simulink model "NandiniG_23EEM1S02_bldc_foc"  (R2024b)
settings: Solver=VariableStepAuto  StartTime=0.0  StopTime=1  FixedStep=0.000001  MaxStep=1e-4  RelTol=1e-3
model workspace (MAT data in the model file):
  fs = 4000
undefined symbols (not defined in the file): Ts
libraries: simulink x13, spsIGBTDiodeLib x6, slpidlib x3, spsPermanentMagnetSynchronousMachineLib x1, spsDCVoltageSourceLib x1, spsSawtoothGeneratorLib x1, simulink_extras x1, spsThreePhaseVIMeasurementLib x1, spspowerguiLib x1
settings Model: Creator=Admin  LastModifiedBy=INNAGOL2
settings SolverCC: ZeroCrossAlgorithm=Adaptive
settings DebuggingCC: MaskedZcDiagnostic=none  IgnoredZcDiagnostic=none
settings RTWCC: GPUComputeCapability=3.5

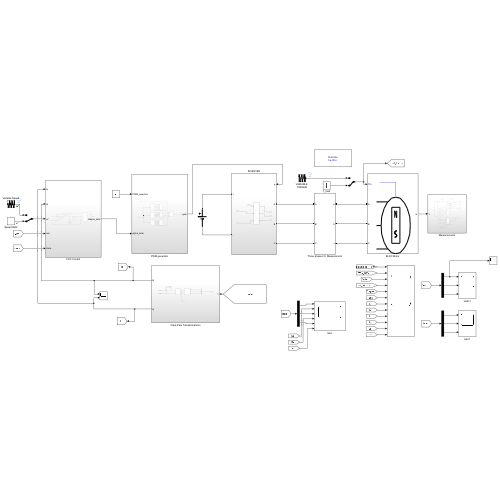
[thumbnail: Simulink's stored preview of the top-level diagram]
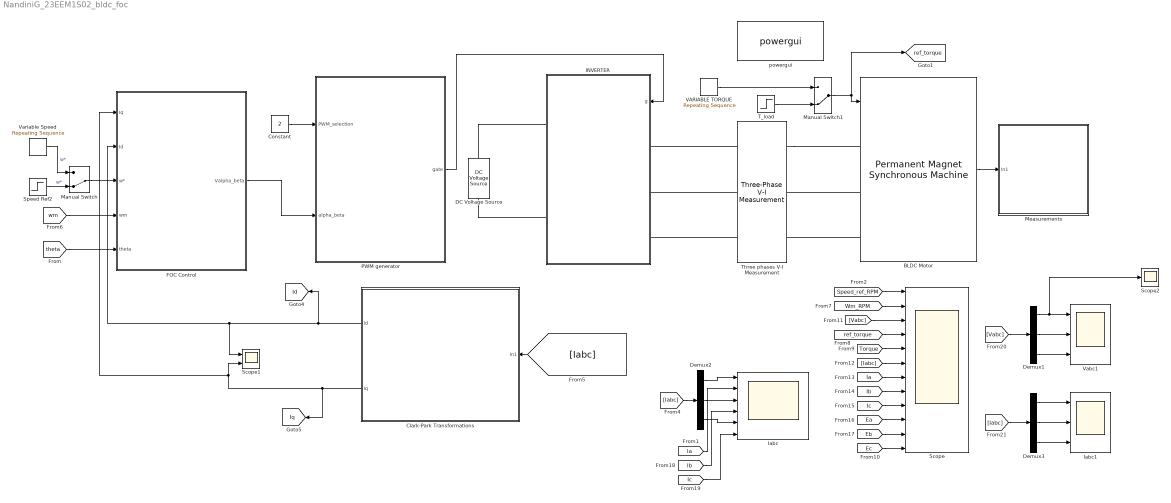
== system NandiniG_23EEM1S02_bldc_foc ==
  BLDC Motor : spsPermanentMagnetSynchronousMachineLib/Permanent Magnet Synchronous Machine  NbPhases=3  FluxDistribution=Trapezoidal  RotorType=Round  MechanicalLoad=Torque Tm  PresetModel=No  ShowDetailedParameters=on  MeasurementBus=off  Resistance=0.7  Inductance=2.7e-3  dqInductances=[8.5e-3,8.5e-3]  La=0.000835  MachineConstant=Flux linkage established by magnets (V.s)  Flux=0.1194  VoltageCst=100.0283  TorqueCst=0.9552  Flat=120  Mechanical=[0.0027 0.0004924 4]  PolePairs=4  InitialConditions=[0,0, 0,0]  InitialConditions5ph=[0 0 0 0 0 0]  RefAngle=Aligned with phase A axis (original Park)  IterativeDiscreteModel=Trapezoidal non iterative  TsBlock=-1  TsPowergui=0
  Clark-Park Transformations : Subsystem
      settings: PortSchema="{\"entries\":[{\"content\":{\"sides\":[{\"content\":{\"connectorIds\":[\"Out1\",\"Out2\"]},\"type\":\"ConnectorPlacement.EquallySpacedRectSide\",\"uuid\":\"c290a13d-b4ce-440f-9d53-4b9274feb83f\"},{\"content\":{\"connectorIds\":[\"In1\"],\"side\":\"RIGHT\"},\"type\":\"ConnectorPlacement.EquallySpacedRectSide\",\"uuid\":\"3b8acf4d-0134-48df-ade6-fa9dd8548719\"},{\"content\":{\"side\":\"TOP\"},\"type\":\"ConnectorPlacement.EquallySpacedRectSide\",\"uuid\":\"08682ee2-bcb7-4f48-a64a-1997ed6d0a04\"}]},\"type\":\"ConnectorPlacement.EquallySpacedConnector\",\"uuid\":\"e640fd84-78ba-4bab-8695-1c4b1b64123a\"}],\"packageUris\":[\"http://schema.mathworks.com/mf0/Connector/R2020b\"],\"version\":\"1.0\"}"
  Constant : Constant  Value=2
  DC Voltage Source : spsDCVoltageSourceLib/DC Voltage Source  Amplitude=160  Measurements=None
  Demux1 : Demux  Outputs=3
  Demux2 : Demux  Outputs=3
  Demux3 : Demux  Outputs=3
  FOC Control : Subsystem
  INVERTER : Subsystem
  Iabc : Scope  NumInputPorts=6
  Iabc1 : Scope  NumInputPorts=3
  Manual Switch : ManualSwitch  CurrentSetting=0
  Manual Switch1 : ManualSwitch  CurrentSetting=0
  Measurements : Subsystem
  PWM generator : Subsystem
  Scope : Scope  NumInputPorts=12
  Scope1 : Scope  NumInputPorts=2
  Scope2 : Scope
  Speed Ref2 : Step  Time=0.1  After=150  SampleTime=0
  "T_load " : Step  Time=0.1  After=5  SampleTime=0
  Three phases V-I Measurement : spsThreePhaseVIMeasurementLib/Three-Phase V-I Measurement  VoltageMeasurement=phase-to-phase  SetLabelV=on  LabelV=Vabc  Vpu=off  VpuLL=off  CurrentMeasurement=yes  SetLabelI=on  LabelI=Iabc  Ipu=off  Pbase=100e6  Vbase=500e3  OutputType=Complex  PhasorSimulation=off  PSBequivalent=0
  VARIABLE TORQUE : simulink/Sources/Repeating Sequence  rep_seq_t=[0 1 2 3 4 5 6 7 8 9 10 11 12 13]  rep_seq_y=[3 3 3 3 5 5 5 -2 -2 -2 1 1 1 1 ]
  Vabc1 : Scope  NumInputPorts=3
  Variable Speed : simulink/Sources/Repeating Sequence  rep_seq_t=[0 1 2 3 4 5 6 7 8 9 10 11 11.0001 12 13]  rep_seq_y=[0 20 20 0 0 0 -30 -30 0 0 50 50 40 40 0]
  powergui : spspowerguiLib/powergui  Priority=1  SimulationMode=Discrete  SampleTime=5e-05  frequency=60  Iterations=50  frequencyindice=0  Pbase=100e6  ErrMax=1e-4  UnitsV=kV  UnitsW=MW  buscounter=0  FunctionMessages=off  echomessages=off  EnableUseOfTLC=off  CurrentSourceSwitches=off  DisableSnubberDevices=off  DisableRonSwitches=off  DisableVfSwitches=off  DisplayEquations=off  AutomaticDiscreteSolvers=off  SolverType=Tustin/Backward Euler (TBE)  Interpol=off  ExternalGateDelay=off  methode=off  Ts=100  x0status=blocks  SPID=on  SwTol=0  HookPort=off  NonlinearTolerance=1e-4  nMaxIteration=100  ContinueOnMaxIteration=off  RestoreLinks=warning  ResistiveCurrentMeasurement=off  Frange=[0:2:500]  Ylog=off  Xlog=on  ShowGrid=off  save=off  variable=ZData  structure=0  ZoomFFT=off  StartTime=0.0  cycles=1  DisplayStyle=1  fundamental=60  FreqAxis=off  MaxFrequency=1000  frequencyindicesteady=1  RmsSteady=1  display=off
  tag scope: Id=global, Iq=global, ref_torque=global
  wires:
  Demux2/1 -> Iabc/1
  Demux2/2 -> Iabc/3
  Demux2/3 -> Iabc/5
  [Iabc] -> Demux2/1
  PWM generator/1(gate) -> INVERTER/1(g)
  [Iabc] -> Clark-Park Transformations/1(In1)
  Clark-Park Transformations/1(Id) -> Scope1/1, FOC Control/2(Id), [Id]
  Clark-Park Transformations/2(Iq) -> Scope1/2, FOC Control/1(Iq), [Iq]
  [wm] -> FOC Control/4(wm)
  [theta] -> FOC Control/5(theta)
  Constant/1 -> PWM generator/1(PWM_selection)
  FOC Control/1(Valpha_beta) -> PWM generator/2(alpha_beta)
  Speed Ref2/1 -> Manual Switch/2  "w*"
  Manual Switch/1 -> FOC Control/3(w*)
  VARIABLE TORQUE/1 -> Manual Switch1/1
  "T_load "/1 -> Manual Switch1/2
  Manual Switch1/1 -> BLDC Motor/1, [ref_torque]
  Variable Speed/1 -> Manual Switch/1  "w*"
  BLDC Motor/1 -> Measurements/1(In1)
  [Vabc] -> Scope/3
  [Ib] -> Scope/8
  [Ia] -> Scope/7
  [Ea] -> Scope/10
  [ref_torque] -> Scope/4
  [Ic] -> Scope/9
  [Ec] -> Scope/12
  [Eb] -> Scope/11
  [Torque] -> Scope/5
  [Wm_RPM] -> Scope/2
  [Iabc] -> Scope/6
  [Speed_ref_RPM] -> Scope/1
  [Ia] -> Iabc/2
  [Ib] -> Iabc/4
  [Ic] -> Iabc/6
  Demux1/2 -> Vabc1/2
  Demux3/2 -> Iabc1/2
  [Vabc] -> Demux1/1
  Demux3/3 -> Iabc1/3
  Demux1/1 -> Scope2/1, Vabc1/1
  Demux1/3 -> Vabc1/3
  Demux3/1 -> Iabc1/1
  [Iabc] -> Demux3/1
  connections:
  BLDC Motor/LConn2 -- Three phases V-I Measurement/RConn2
  BLDC Motor/LConn3 -- Three phases V-I Measurement/RConn3
  Three phases V-I Measurement/LConn1 -- INVERTER/LConn1
  DC Voltage Source/RConn1 -- INVERTER/RConn1
  Three phases V-I Measurement/LConn2 -- INVERTER/LConn2
  DC Voltage Source/LConn1 -- INVERTER/RConn2
  Three phases V-I Measurement/LConn3 -- INVERTER/LConn3
  Three phases V-I Measurement/RConn1 -- BLDC Motor/LConn1

== system NandiniG_23EEM1S02_bldc_foc/Clark-Park Transformations ==
  In1 : Inport
  Clark Transformation : Subsystem
  Demux1 : Demux  Outputs=3
  Park Transformation : Subsystem
  Scope3 : Scope  NumInputPorts=2
  Id : Outport
  Iq : Outport  Port=2
  wires:
  Park Transformation/2(Iq) -> Iq/1, Scope3/2  "Iq"
  Demux1/1 -> Clark Transformation/1(Ia)
  Park Transformation/1(Id) -> Id/1, Scope3/1  "Id"
  [theta] -> Park Transformation/3(theta)
  Demux1/2 -> Clark Transformation/2(Ib)
  Clark Transformation/2(I_beta) -> Park Transformation/2(I_beta)
  Demux1/3 -> Clark Transformation/3(Ic)
  Clark Transformation/1(I_alpha) -> Park Transformation/1(I_alpha)
  In1/1 -> Demux1/1

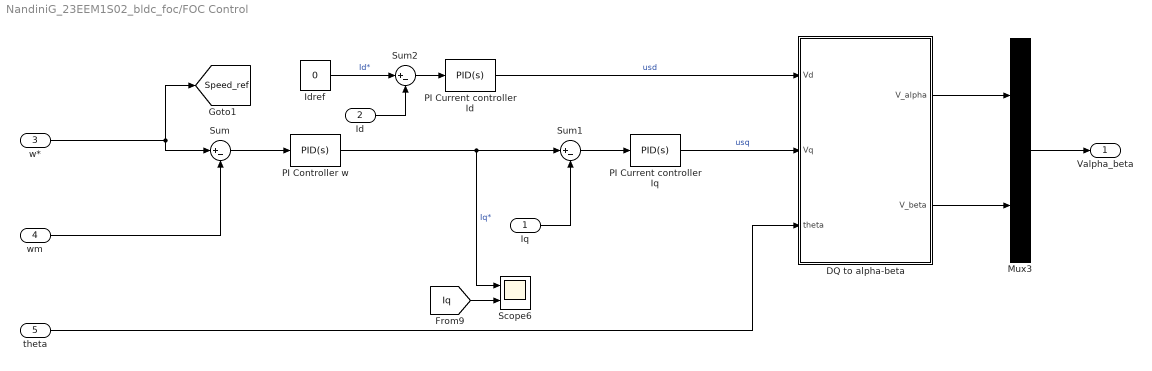
== system NandiniG_23EEM1S02_bldc_foc/FOC Control ==
  Iq : Inport
  Id : Inport  Port=2
  w* : Inport  Port=3
  wm : Inport  Port=4
  theta : Inport  Port=5
  DQ to alpha-beta : Subsystem
  Idref : Constant  Value=0
  Mux3 : Mux  Inputs=2
  PI Controller w : slpidlib/PID Controller  Controller=PID  Form=Parallel  TimeDomain=Continuous-time  UseExternalTs=off  SampleTime=-1  IntegratorMethod=Forward Euler  FilterMethod=Forward Euler  ControllerParametersSource=internal  P=18  I=35  UseKiTs=off  D=0  UseExternalDerivativeSource=off  N=100  UseFilter=on  TunerSelectOption=Frequency Response Based  InitialConditionSource=internal  InitialConditionForIntegrator=0  InitialConditionForFilter=0  DifferentiatorICPrevScaledInput=0  ExternalReset=none  TrackingMode=off  Kt=1  LimitOutput=on  SatLimitsSource=internal  UpperSaturationLimit=60  LowerSaturationLimit=-60  LinearizeAsGain=on  AntiWindupMode=none  Kb=1  LimitIntegrator=on  UpperIntegratorSaturationLimit=60  LowerIntegratorSaturationLimit=-60  POutMin=[]  POutMax=[]  IOutMin=[]  IOutMax=[]  DOutMin=[]  DOutMax=[]  NOutMin=[]  NOutMax=[]  SumOutMin=[]  SumOutMax=[]  SaturationOutMin=[]  SaturationOutMax=[]  PParamMin=[]  PParamMax=[]  IParamMin=[]  IParamMax=[]  DParamMin=[]  DParamMax=[]  NParamMin=[]  NParamMax=[]  KbParamMin=[]  KbParamMax=[]  KtParamMin=[]  KtParamMax=[]  KbOutMin=[]  KbOutMax=[]  KtOutMin=[]  KtOutMax=[]  IntegratorOutMin=[]  IntegratorOutMax=[]  FilterOutMin=[]  FilterOutMax=[]  SumI1OutMin=[]  SumI1OutMax=[]  SumI2OutMin=[]  SumI2OutMax=[]  SumI3OutMin=[]  SumI3OutMax=[]  SumI4OutMin=[]  SumI4OutMax=[]  SumDOutMin=[]  SumDOutMax=[]  DifferentiatorOutMin=[]  DifferentiatorOutMax=[]  FilterDiffOutCoefMin=[]  FilterDiffOutCoefMax=[]  ReciprocalOutMin=[]  ReciprocalOutMax=[]  SumDenOutMin=[]  SumDenOutMax=[]  SumNumOutMin=[]  SumNumOutMax=[]  DivideOutMin=[]  DivideOutMax=[]  UdiffTsProdOutMin=[]  UdiffTsProdOutMax=[]  NTsProdOutMin=[]  NTsProdOutMax=[]  UintegralTsProdOutMin=[]  UintegralTsProdOutMax=[]  UngainTsProdOutMin=[]  UngainTsProdOutMax=[]  ClampingZeroOutDataTypeStr=Inherit: Inherit via back propagation  ClampingZeroOutMin=[]  ClampingZeroOutMax=[]  FilterDenConstantOutDataTypeStr=Inherit: Inherit via back propagation  FilterDenConstantOutMin=[]  FilterDenConstantOutMax=[]  PCopyOutDataTypeStr=Inherit: Inherit via back propagation  PCopyOutMin=[]  PCopyOutMax=[]  NCopyOutDataTypeStr=Inherit: Inherit via back propagation  NCopyOutMin=[]  NCopyOutMax=[]  IntegratorContinuousStateAttributes=''  IntegratorStateMustResolveToSignalObject=off  IntegratorRTWStateStorageClass=Auto  FilterContinuousStateAttributes=''  FilterStateMustResolveToSignalObject=off  FilterRTWStateStorageClass=Auto  ParallelPVariant=InternalParameters  IdealPVariant=Disabled  IVariant=InternalParameters  DVariant=InternalParameters  IntegratorVariant=Continuous  SatVariant=Enabled  AWVariant=Passthrough  PCopyVariant=Disabled  TRVariant=Disabled  FdbkBlocksVariant=Forward  IdealPFdbkVariant=Disabled  SatFdbkVariant=Disabled  DerivativeFilterVariant=ContFilter  NVariant=InternalParameters  NCopyVariant=Disabled  FilterICVariant=InternalICsFilter  IntegratorICVariant=InternalICs  ExternalResetVariant=Disabled  TRSumVariant=Passthrough  SumFdbkVariant=Disabled  SumVariant=Sum_PID  TsampFilterVariant=InternalTs  TsampNgainVariant=Passthrough  TsampIntegralVariant=Disabled_SignalSpec  ExternalSaturationOutDataTypeStr=Inherit: Same as second input  DerivativeSourceVariant=ErrorSignal  PreIntVariant=InternalPreInt
  PI Current controller Id : slpidlib/PID Controller  Controller=PID  Form=Parallel  TimeDomain=Continuous-time  UseExternalTs=off  SampleTime=-1  IntegratorMethod=Forward Euler  FilterMethod=Forward Euler  ControllerParametersSource=internal  P=100  I=1000  UseKiTs=off  D=0  UseExternalDerivativeSource=off  N=100  UseFilter=on  TunerSelectOption=Transfer Function Based (PID Tuner App)  InitialConditionSource=internal  InitialConditionForIntegrator=0  InitialConditionForFilter=0  DifferentiatorICPrevScaledInput=0  ExternalReset=none  TrackingMode=off  Kt=1  LimitOutput=on  SatLimitsSource=internal  UpperSaturationLimit=600  LowerSaturationLimit=-600  LinearizeAsGain=on  AntiWindupMode=clamping  Kb=1  LimitIntegrator=off  UpperIntegratorSaturationLimit=inf  LowerIntegratorSaturationLimit=-inf  POutMin=[]  POutMax=[]  IOutMin=[]  IOutMax=[]  DOutMin=[]  DOutMax=[]  NOutMin=[]  NOutMax=[]  SumOutMin=[]  SumOutMax=[]  SaturationOutMin=[]  SaturationOutMax=[]  PParamMin=[]  PParamMax=[]  IParamMin=[]  IParamMax=[]  DParamMin=[]  DParamMax=[]  NParamMin=[]  NParamMax=[]  KbParamMin=[]  KbParamMax=[]  KtParamMin=[]  KtParamMax=[]  KbOutMin=[]  KbOutMax=[]  KtOutMin=[]  KtOutMax=[]  IntegratorOutMin=[]  IntegratorOutMax=[]  FilterOutMin=[]  FilterOutMax=[]  SumI1OutMin=[]  SumI1OutMax=[]  SumI2OutMin=[]  SumI2OutMax=[]  SumI3OutMin=[]  SumI3OutMax=[]  SumI4OutMin=[]  SumI4OutMax=[]  SumDOutMin=[]  SumDOutMax=[]  DifferentiatorOutMin=[]  DifferentiatorOutMax=[]  FilterDiffOutCoefMin=[]  FilterDiffOutCoefMax=[]  ReciprocalOutMin=[]  ReciprocalOutMax=[]  SumDenOutMin=[]  SumDenOutMax=[]  SumNumOutMin=[]  SumNumOutMax=[]  DivideOutMin=[]  DivideOutMax=[]  UdiffTsProdOutMin=[]  UdiffTsProdOutMax=[]  NTsProdOutMin=[]  NTsProdOutMax=[]  UintegralTsProdOutMin=[]  UintegralTsProdOutMax=[]  UngainTsProdOutMin=[]  UngainTsProdOutMax=[]  ClampingZeroOutDataTypeStr=Inherit: Inherit via back propagation  ClampingZeroOutMin=[]  ClampingZeroOutMax=[]  FilterDenConstantOutDataTypeStr=Inherit: Inherit via back propagation  FilterDenConstantOutMin=[]  FilterDenConstantOutMax=[]  PCopyOutDataTypeStr=Inherit: Inherit via back propagation  PCopyOutMin=[]  PCopyOutMax=[]  NCopyOutDataTypeStr=Inherit: Inherit via back propagation  NCopyOutMin=[]  NCopyOutMax=[]  IntegratorContinuousStateAttributes=''  IntegratorStateMustResolveToSignalObject=off  IntegratorRTWStateStorageClass=Auto  FilterContinuousStateAttributes=''  FilterStateMustResolveToSignalObject=off  FilterRTWStateStorageClass=Auto  ParallelPVariant=InternalParameters  IdealPVariant=Disabled  IVariant=InternalParameters  DVariant=InternalParameters  IntegratorVariant=Continuous  SatVariant=Enabled  AWVariant=ContClampingParallel  PCopyVariant=Disabled  TRVariant=Disabled  FdbkBlocksVariant=Forward  IdealPFdbkVariant=Disabled  SatFdbkVariant=Disabled  DerivativeFilterVariant=ContFilter  NVariant=InternalParameters  NCopyVariant=Disabled  FilterICVariant=InternalICsFilter  IntegratorICVariant=InternalICs  ExternalResetVariant=Disabled  TRSumVariant=Passthrough  SumFdbkVariant=Disabled  SumVariant=Sum_PID  TsampFilterVariant=InternalTs  TsampNgainVariant=Passthrough  TsampIntegralVariant=Disabled_SignalSpec  ExternalSaturationOutDataTypeStr=Inherit: Same as second input  DerivativeSourceVariant=ErrorSignal  PreIntVariant=InternalPreInt
  PI Current controller Iq : slpidlib/PID Controller  Controller=PID  Form=Parallel  TimeDomain=Continuous-time  UseExternalTs=off  SampleTime=-1  IntegratorMethod=Forward Euler  FilterMethod=Forward Euler  ControllerParametersSource=internal  P=100  I=1000  UseKiTs=off  D=0  UseExternalDerivativeSource=off  N=100  UseFilter=on  TunerSelectOption=Transfer Function Based (PID Tuner App)  InitialConditionSource=internal  InitialConditionForIntegrator=0  InitialConditionForFilter=0  DifferentiatorICPrevScaledInput=0  ExternalReset=none  TrackingMode=off  Kt=1  LimitOutput=on  SatLimitsSource=internal  UpperSaturationLimit=600  LowerSaturationLimit=-600  LinearizeAsGain=on  AntiWindupMode=clamping  Kb=1  LimitIntegrator=off  UpperIntegratorSaturationLimit=inf  LowerIntegratorSaturationLimit=-inf  POutMin=[]  POutMax=[]  IOutMin=[]  IOutMax=[]  DOutMin=[]  DOutMax=[]  NOutMin=[]  NOutMax=[]  SumOutMin=[]  SumOutMax=[]  SaturationOutMin=[]  SaturationOutMax=[]  PParamMin=[]  PParamMax=[]  IParamMin=[]  IParamMax=[]  DParamMin=[]  DParamMax=[]  NParamMin=[]  NParamMax=[]  KbParamMin=[]  KbParamMax=[]  KtParamMin=[]  KtParamMax=[]  KbOutMin=[]  KbOutMax=[]  KtOutMin=[]  KtOutMax=[]  IntegratorOutMin=[]  IntegratorOutMax=[]  FilterOutMin=[]  FilterOutMax=[]  SumI1OutMin=[]  SumI1OutMax=[]  SumI2OutMin=[]  SumI2OutMax=[]  SumI3OutMin=[]  SumI3OutMax=[]  SumI4OutMin=[]  SumI4OutMax=[]  SumDOutMin=[]  SumDOutMax=[]  DifferentiatorOutMin=[]  DifferentiatorOutMax=[]  FilterDiffOutCoefMin=[]  FilterDiffOutCoefMax=[]  ReciprocalOutMin=[]  ReciprocalOutMax=[]  SumDenOutMin=[]  SumDenOutMax=[]  SumNumOutMin=[]  SumNumOutMax=[]  DivideOutMin=[]  DivideOutMax=[]  UdiffTsProdOutMin=[]  UdiffTsProdOutMax=[]  NTsProdOutMin=[]  NTsProdOutMax=[]  UintegralTsProdOutMin=[]  UintegralTsProdOutMax=[]  UngainTsProdOutMin=[]  UngainTsProdOutMax=[]  ClampingZeroOutDataTypeStr=Inherit: Inherit via back propagation  ClampingZeroOutMin=[]  ClampingZeroOutMax=[]  FilterDenConstantOutDataTypeStr=Inherit: Inherit via back propagation  FilterDenConstantOutMin=[]  FilterDenConstantOutMax=[]  PCopyOutDataTypeStr=Inherit: Inherit via back propagation  PCopyOutMin=[]  PCopyOutMax=[]  NCopyOutDataTypeStr=Inherit: Inherit via back propagation  NCopyOutMin=[]  NCopyOutMax=[]  IntegratorContinuousStateAttributes=''  IntegratorStateMustResolveToSignalObject=off  IntegratorRTWStateStorageClass=Auto  FilterContinuousStateAttributes=''  FilterStateMustResolveToSignalObject=off  FilterRTWStateStorageClass=Auto  ParallelPVariant=InternalParameters  IdealPVariant=Disabled  IVariant=InternalParameters  DVariant=InternalParameters  IntegratorVariant=Continuous  SatVariant=Enabled  AWVariant=ContClampingParallel  PCopyVariant=Disabled  TRVariant=Disabled  FdbkBlocksVariant=Forward  IdealPFdbkVariant=Disabled  SatFdbkVariant=Disabled  DerivativeFilterVariant=ContFilter  NVariant=InternalParameters  NCopyVariant=Disabled  FilterICVariant=InternalICsFilter  IntegratorICVariant=InternalICs  ExternalResetVariant=Disabled  TRSumVariant=Passthrough  SumFdbkVariant=Disabled  SumVariant=Sum_PID  TsampFilterVariant=InternalTs  TsampNgainVariant=Passthrough  TsampIntegralVariant=Disabled_SignalSpec  ExternalSaturationOutDataTypeStr=Inherit: Same as second input  DerivativeSourceVariant=ErrorSignal  PreIntVariant=InternalPreInt
  Scope6 : Scope  NumInputPorts=2
  Sum : Sum  Inputs=|+-
  Sum1 : Sum  Inputs=|+-
  Sum2 : Sum  Inputs=|+-
  Valpha_beta : Outport
  tag scope: Speed_ref=global
  wires:
  PI Current controller Iq/1 -> DQ to alpha-beta/2(Vq)  "usq"
  PI Controller w/1 -> Scope6/1, Sum1/1  "Iq*"
  theta/1 -> DQ to alpha-beta/3(theta)
  Idref/1 -> Sum2/1  "Id*"
  Sum1/1 -> PI Current controller Iq/1
  Sum2/1 -> PI Current controller Id/1
  Sum/1 -> PI Controller w/1
  w*/1 -> [Speed_ref], Sum/1
  [Iq] -> Scope6/2
  PI Current controller Id/1 -> DQ to alpha-beta/1(Vd)  "usd"
  DQ to alpha-beta/1(V_alpha) -> Mux3/1
  DQ to alpha-beta/2(V_beta) -> Mux3/2
  Mux3/1 -> Valpha_beta/1
  Iq/1 -> Sum1/2
  wm/1 -> Sum/2
  Id/1 -> Sum2/2

== system NandiniG_23EEM1S02_bldc_foc/INVERTER ==
  g : Inport
  Subsystem1 : Subsystem
  A : PMIOPort  Side=Left
  B : PMIOPort  Port=2  Side=Left
  C : PMIOPort  Port=3  Side=Left
  + : PMIOPort  Port=4  Side=Right
  - : PMIOPort  Port=5  Side=Right
  wires:
  g/1 -> Subsystem1/1(Gate)
  connections:
  C/RConn1 -- Subsystem1/RConn3
  B/RConn1 -- Subsystem1/RConn2
  A/RConn1 -- Subsystem1/RConn1
  +/RConn1 -- Subsystem1/LConn1
  -/RConn1 -- Subsystem1/LConn2

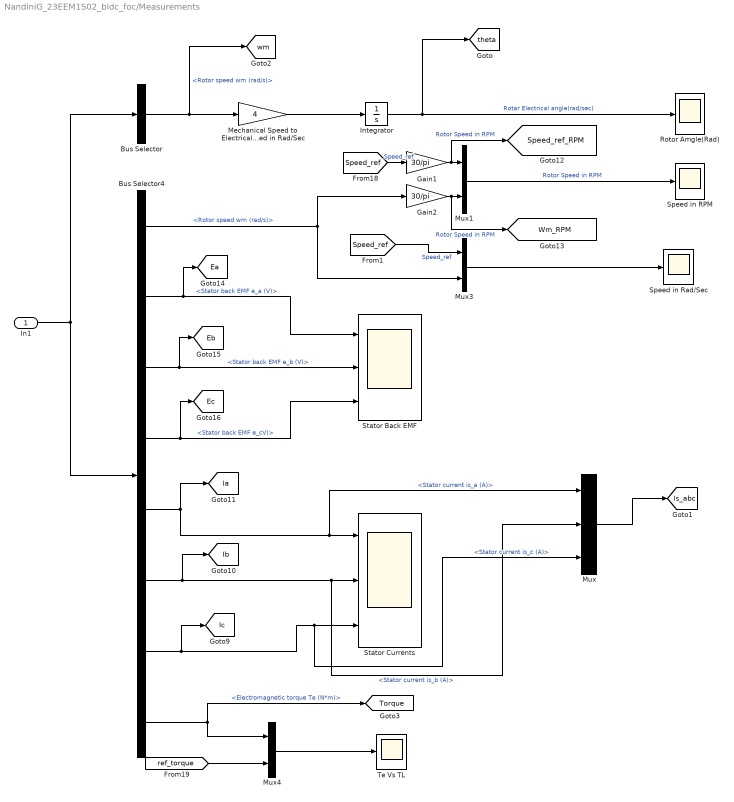
== system NandiniG_23EEM1S02_bldc_foc/Measurements ==
  In1 : Inport
  Bus Selector : BusSelector  OutputSignals=Rotor speed wm (rad/s)
  Bus Selector4 : BusSelector  OutputSignals=Rotor speed wm (rad/s),Stator back EMF e_a (V),Stator back EMF e_b (V),Stator back EMF e_cV),Stator current is_a (A),Stator current is_b (A),Stator current is_c (A),Electromagnetic torque Te (N*m)
  Gain1 : Gain  Gain=30/pi
  Gain2 : Gain  Gain=30/pi
  Integrator : Integrator  WrapState=on
  Mechanical Speed to Electrical speed in Rad/Sec : Gain  Gain=4
  Mux : Mux  Inputs=3
  Mux1 : Mux  Inputs=2
  Mux3 : Mux  Inputs=2
  Mux4 : Mux  Inputs=2
  Rotor Amgle(Rad) : Scope
  Speed in RPM : Scope
  Speed in Rad/Sec : Scope
  Stator Back EMF : Scope  NumInputPorts=3
  Stator Currents : Scope  NumInputPorts=3
  Te Vs TL : Scope
  tag scope: Ea=global, Eb=global, Ec=global, Ia=global, Ib=global, Ic=global, Is_abc=global, Speed_ref_RPM=global, Torque=global, Wm_RPM=global, theta=global, wm=global
  wires:
  [ref_torque] -> Mux4/2
  Mechanical Speed to Electrical speed in Rad/Sec/1 -> Integrator/1
  Mux4/1 -> Te Vs TL/1
  Bus Selector/1 -> [wm], Mechanical Speed to Electrical speed in Rad/Sec/1  "<Rotor speed wm (rad/s)>"
  Bus Selector4/3 -> [Eb], Stator Back EMF/2  "<Stator back EMF e_b (V)>"
  Bus Selector4/8 -> [Torque], Mux4/1  "<Electromagnetic torque Te (N*m)>"
  Bus Selector4/5 -> [Ia], Mux/1, Stator Currents/1  "<Stator current is_a (A)>"
  In1/1 -> Bus Selector4/1, Bus Selector/1
  Bus Selector4/4 -> [Ec], Stator Back EMF/3  "<Stator back EMF e_cV)>"
  Gain2/1 -> [Wm_RPM], Mux1/2  "Rotor Speed in RPM"
  Bus Selector4/7 -> [Ic], Mux/3, Stator Currents/3  "<Stator current is_c (A)>"
  Integrator/1 -> [theta], Rotor Amgle(Rad)/1  "Rotar Electrical angle(rad/sec)"
  Bus Selector4/2 -> [Ea], Stator Back EMF/1  "<Stator back EMF e_a (V)>"
  Bus Selector4/1 -> Mux3/2, Gain2/1  "<Rotor speed wm (rad/s)>"
  Gain1/1 -> [Speed_ref_RPM], Mux1/1  "Rotor Speed in RPM"
  Mux3/1 -> Speed in Rad/Sec/1
  Mux1/1 -> Speed in RPM/1  "Rotor Speed in RPM"
  [Speed_ref] -> Gain1/1  "Speed_ref"
  Bus Selector4/6 -> [Ib], Mux/2, Stator Currents/2  "<Stator current is_b (A)>"
  [Speed_ref] -> Mux3/1  "Speed_ref"
  Mux/1 -> [Is_abc]

== system NandiniG_23EEM1S02_bldc_foc/PWM generator ==
  PWM_selection : Inport
  alpha_beta : Inport  Port=2
  Gate : Scope  NumInputPorts=6
  Multiport Switch : MultiPortSwitch  SaturateOnIntegerOverflow=off  InputSameDT=off
  PWM : Subsystem
  SPWM : Subsystem
  SVPWM : Subsystem
  Scope4 : Scope  NumInputPorts=6
  Scope9 : Scope  NumInputPorts=6
  gate : Outport
  wires:
  SVPWM/2(g4) -> Scope9/2
  PWM/2(g4) -> Scope4/2
  PWM/3(g3) -> Scope4/3
  PWM/1(g1) -> Scope4/1
  SPWM/3(g3) -> Gate/3
  SVPWM/1(g1) -> Scope9/1
  alpha_beta/1 -> SPWM/1(alpha_beta), SVPWM/1(alpha beta), PWM/1(alpha_beta)
  SVPWM/3(g3) -> Scope9/3
  PWM/5(g5) -> Scope4/5
  PWM/7(Gate) -> Multiport Switch/4
  PWM/6(g2) -> Scope4/6
  SPWM/5(g5) -> Gate/5
  SPWM/4(g6) -> Gate/4
  SPWM/1(g1) -> Gate/1
  SPWM/2(g4) -> Gate/2
  SPWM/6(g2) -> Gate/6
  SPWM/7(gate) -> Multiport Switch/2
  PWM/4(g6) -> Scope4/4
  PWM_selection/1 -> Multiport Switch/1
  Multiport Switch/1 -> gate/1
  SVPWM/4(g6) -> Scope9/4
  SVPWM/5(g5) -> Scope9/5
  SVPWM/6(g2) -> Scope9/6
  SVPWM/7(Gate1) -> Multiport Switch/3

== system NandiniG_23EEM1S02_bldc_foc/Clark-Park Transformations/Clark Transformation ==
  Ia : Inport
  Ib : Inport  Port=2
  Ic : Inport  Port=3
  Gain : Gain
  Gain1 : Gain  Gain=-1/2
  Gain2 : Gain  Gain=-1/2
  Gain3 : Gain  Gain=(sqrt(3))/2
  Gain4 : Gain  Gain=(-sqrt(3))/2
  Sum3 : Sum  Inputs=|+++
  Sum4 : Sum  Inputs=|++
  I_alpha : Outport
  I_beta : Outport  Port=2
  wires:
  Gain2/1 -> Sum3/3
  Ib/1 -> Gain3/1, Gain1/1
  Sum3/1 -> I_alpha/1
  Gain3/1 -> Sum4/1
  Gain/1 -> Sum3/1
  Ic/1 -> Gain4/1, Gain2/1
  Gain1/1 -> Sum3/2
  Gain4/1 -> Sum4/2
  Ia/1 -> Gain/1
  Sum4/1 -> I_beta/1

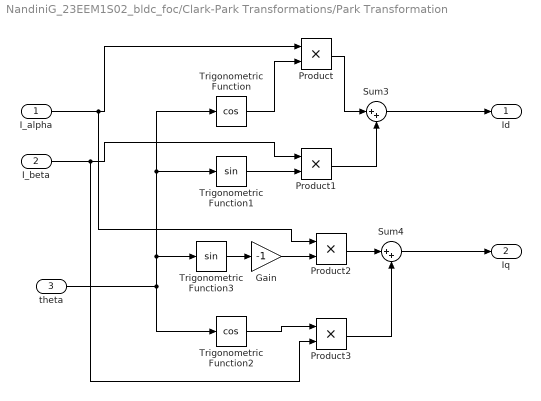
== system NandiniG_23EEM1S02_bldc_foc/Clark-Park Transformations/Park Transformation ==
  I_alpha : Inport
  I_beta : Inport  Port=2
  theta : Inport  Port=3
  Gain : Gain  Gain=-1
  Product{,1..3} (4 alike) : Product
  Sum3 : Sum  Inputs=|++
  Sum4 : Sum  Inputs=|++
  Trigonometric Function : Trigonometry  Operator=cos
  Trigonometric Function1 : Trigonometry
  Trigonometric Function2 : Trigonometry  Operator=cos
  Trigonometric Function3 : Trigonometry
  Id : Outport
  Iq : Outport  Port=2
  wires:
  Sum3/1 -> Id/1
  Sum4/1 -> Iq/1
  Trigonometric Function3/1 -> Gain/1
  theta/1 -> Trigonometric Function2/1, Trigonometric Function3/1, Trigonometric Function1/1, Trigonometric Function/1
  Trigonometric Function/1 -> Product/2
  I_alpha/1 -> Product2/1, Product/1
  Trigonometric Function1/1 -> Product1/2
  I_beta/1 -> Product3/2, Product1/1
  Product/1 -> Sum3/1
  Product1/1 -> Sum3/2
  Gain/1 -> Product2/2
  Trigonometric Function2/1 -> Product3/1
  Product2/1 -> Sum4/1
  Product3/1 -> Sum4/2

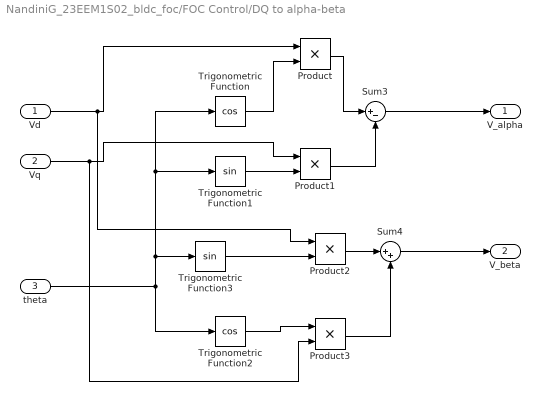
== system NandiniG_23EEM1S02_bldc_foc/FOC Control/DQ to alpha-beta ==
  Vd : Inport
  Vq : Inport  Port=2
  theta : Inport  Port=3
  Product{,1..3} (4 alike) : Product
  Sum3 : Sum  Inputs=|+-
  Sum4 : Sum  Inputs=|++
  Trigonometric Function : Trigonometry  Operator=cos
  Trigonometric Function1 : Trigonometry
  Trigonometric Function2 : Trigonometry  Operator=cos
  Trigonometric Function3 : Trigonometry
  V_alpha : Outport
  V_beta : Outport  Port=2
  wires:
  Product3/1 -> Sum4/2
  Product2/1 -> Sum4/1
  Trigonometric Function2/1 -> Product3/1
  Trigonometric Function3/1 -> Product2/2
  Product1/1 -> Sum3/2
  Product/1 -> Sum3/1
  Vq/1 -> Product1/1, Product3/2
  Trigonometric Function1/1 -> Product1/2
  Vd/1 -> Product/1, Product2/1
  Trigonometric Function/1 -> Product/2
  theta/1 -> Trigonometric Function/1, Trigonometric Function1/1, Trigonometric Function3/1, Trigonometric Function2/1
  Sum4/1 -> V_beta/1
  Sum3/1 -> V_alpha/1

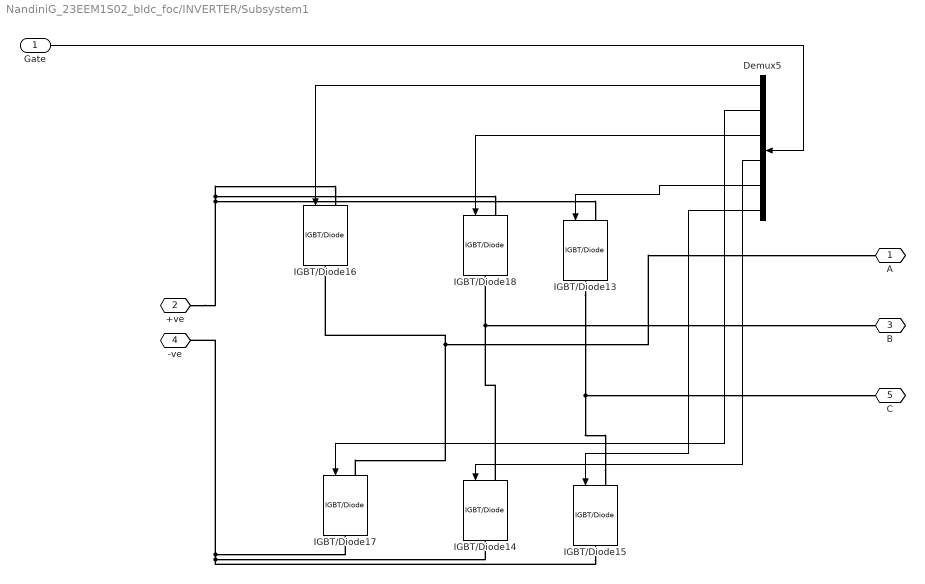
== system NandiniG_23EEM1S02_bldc_foc/INVERTER/Subsystem1 ==
  Gate : Inport
  Demux5 : Demux  Outputs=6
  IGBT/Diode{13..18} (6 alike) : spsIGBTDiodeLib/IGBT//Diode  Ron=1e-3  Rs=1e5  Cs=inf  Measurements=off
  A : PMIOPort  Side=Right
  +ve : PMIOPort  Port=2  Side=Left
  B : PMIOPort  Port=3  Side=Right
  -ve : PMIOPort  Port=4  Side=Left
  C : PMIOPort  Port=5  Side=Right
  wires:
  Demux5/3 -> IGBT/Diode18/1
  Demux5/2 -> IGBT/Diode17/1
  Demux5/6 -> IGBT/Diode15/1
  Demux5/1 -> IGBT/Diode16/1
  Gate/1 -> Demux5/1
  Demux5/4 -> IGBT/Diode14/1
  Demux5/5 -> IGBT/Diode13/1
  connections:
  IGBT/Diode15/LConn1 -- C/RConn1 -- IGBT/Diode13/RConn1
  IGBT/Diode18/RConn1 -- B/RConn1 -- IGBT/Diode14/LConn1
  IGBT/Diode14/RConn1 -- IGBT/Diode17/RConn1 -- -ve/RConn1 -- IGBT/Diode15/RConn1
  IGBT/Diode16/RConn1 -- A/RConn1 -- IGBT/Diode17/LConn1
  IGBT/Diode16/LConn1 -- IGBT/Diode18/LConn1 -- +ve/RConn1 -- IGBT/Diode13/LConn1

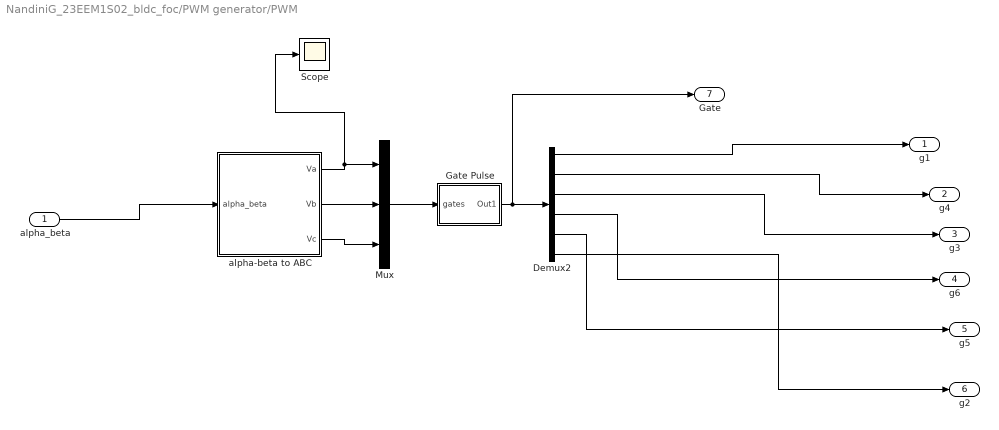
== system NandiniG_23EEM1S02_bldc_foc/PWM generator/PWM ==
  alpha_beta : Inport
  Demux2 : Demux  Outputs=6
  Gate Pulse : Subsystem
  Mux : Mux  Inputs=3
  Scope : Scope
  alpha-beta to ABC : Subsystem
  g1 : Outport
  g4 : Outport  Port=2
  g3 : Outport  Port=3
  g6 : Outport  Port=4
  g5 : Outport  Port=5
  g2 : Outport  Port=6
  Gate : Outport  Port=7
  wires:
  Gate Pulse/1(Out1) -> Gate/1, Demux2/1
  alpha-beta to ABC/3(Vc) -> Mux/3
  Demux2/3 -> g3/1
  alpha-beta to ABC/1(Va) -> Scope/1, Mux/1
  Mux/1 -> Gate Pulse/1(gates)
  Demux2/5 -> g5/1
  Demux2/2 -> g4/1
  alpha-beta to ABC/2(Vb) -> Mux/2
  alpha_beta/1 -> alpha-beta to ABC/1(alpha_beta)
  Demux2/6 -> g2/1
  Demux2/4 -> g6/1
  Demux2/1 -> g1/1

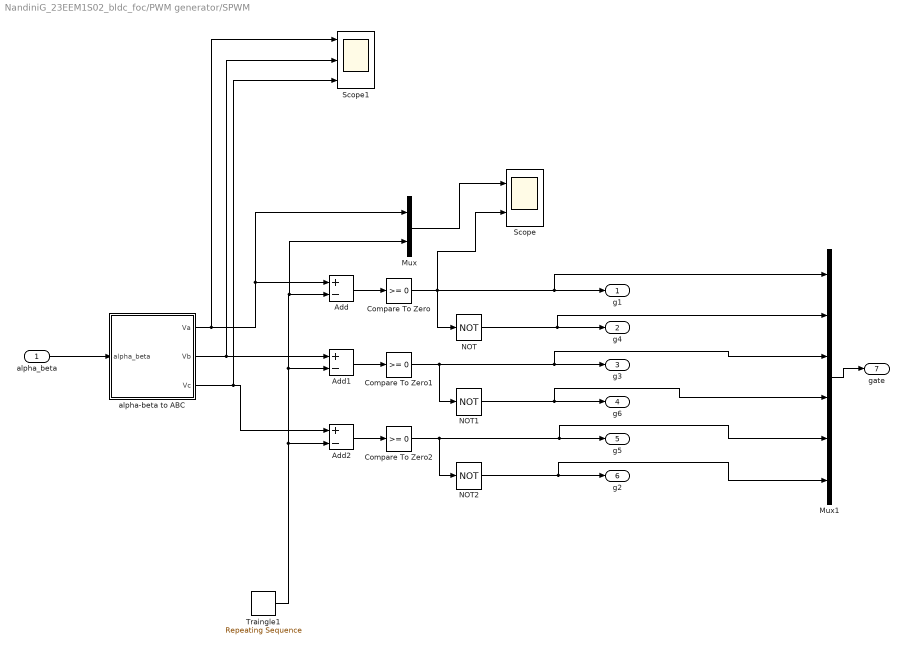
== system NandiniG_23EEM1S02_bldc_foc/PWM generator/SPWM ==
  alpha_beta : Inport
  Add : Sum  Inputs=+-
  Add1 : Sum  Inputs=+-
  Add2 : Sum  Inputs=+-
  Compare To Zero : simulink/Logic and Bit Operations/Compare To Zero  relop=>=  OutDataTypeStr=boolean
  Compare To Zero1 : simulink/Logic and Bit Operations/Compare To Zero  relop=>=  OutDataTypeStr=boolean
  Compare To Zero2 : simulink/Logic and Bit Operations/Compare To Zero  relop=>=  OutDataTypeStr=boolean
  Mux : Mux  Inputs=2
  Mux1 : Mux  Inputs=6
  NOT : Logic  Operator=NOT  AllPortsSameDT=off  OutDataTypeStr=boolean
  NOT1 : Logic  Operator=NOT  AllPortsSameDT=off  OutDataTypeStr=boolean
  NOT2 : Logic  Operator=NOT  AllPortsSameDT=off  OutDataTypeStr=boolean
  Scope : Scope  NumInputPorts=2
  Scope1 : Scope  NumInputPorts=3
  Traingle1 : simulink/Sources/Repeating Sequence  rep_seq_t=[0 1/20000]  rep_seq_y=[-100 100]
  alpha-beta to ABC : Subsystem
  g1 : Outport
  g4 : Outport  Port=2
  g3 : Outport  Port=3
  g6 : Outport  Port=4
  g5 : Outport  Port=5
  g2 : Outport  Port=6
  gate : Outport  Port=7
  wires:
  Compare To Zero2/1 -> Mux1/5, g5/1, NOT2/1
  Compare To Zero/1 -> Mux1/1, g1/1, Scope/2, NOT/1
  Mux/1 -> Scope/1
  alpha-beta to ABC/1(Va) -> Scope1/1, Mux/1, Add/1
  Add/1 -> Compare To Zero/1
  Add2/1 -> Compare To Zero2/1
  Compare To Zero1/1 -> Mux1/3, g3/1, NOT1/1
  Traingle1/1 -> Mux/2, Add/2, Add1/2, Add2/2
  Add1/1 -> Compare To Zero1/1
  alpha_beta/1 -> alpha-beta to ABC/1(alpha_beta)
  NOT1/1 -> Mux1/4, g6/1
  alpha-beta to ABC/2(Vb) -> Scope1/2, Add1/1
  alpha-beta to ABC/3(Vc) -> Scope1/3, Add2/1
  NOT/1 -> Mux1/2, g4/1
  NOT2/1 -> Mux1/6, g2/1
  Mux1/1 -> gate/1

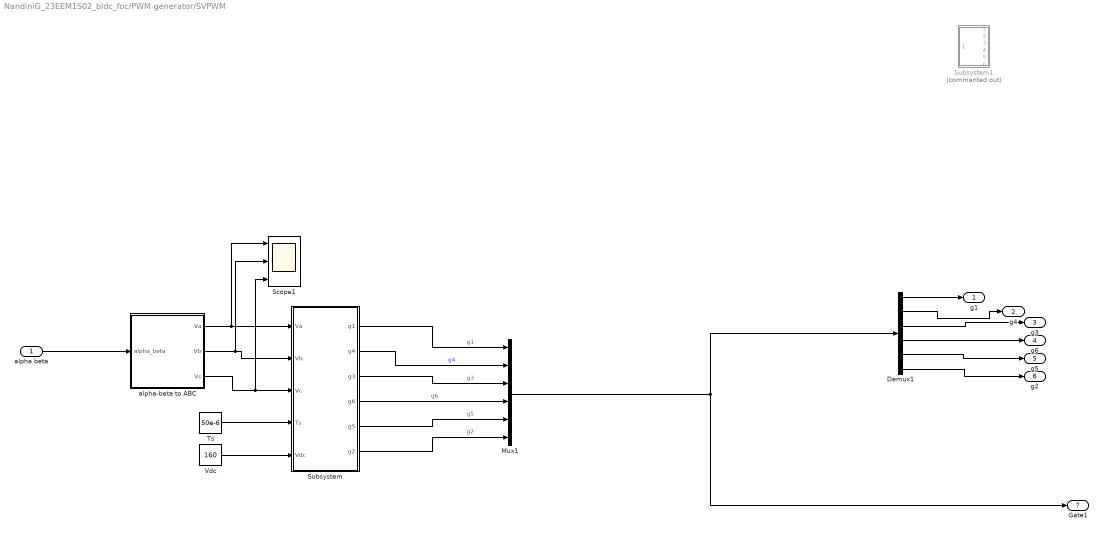
== system NandiniG_23EEM1S02_bldc_foc/PWM generator/SVPWM ==
  alpha beta : Inport
  Demux1 : Demux  Outputs=6
  Mux1 : Mux  Inputs=6
  Scope1 : Scope  NumInputPorts=3
  Subsystem : Subsystem
  Subsystem1 : Subsystem  Commented=on
  Ts : Constant  Value=50e-6
  Vdc : Constant  Value=160
  alpha-beta to ABC : Subsystem
  g1 : Outport
  g4 : Outport  Port=2
  g3 : Outport  Port=3
  g6 : Outport  Port=4
  g5 : Outport  Port=5
  g2 : Outport  Port=6
  Gate1 : Outport  Port=7
  wires:
  Vdc/1 -> Subsystem/5(Vdc)
  Ts/1 -> Subsystem/4(Ts)
  alpha beta/1 -> alpha-beta to ABC/1(alpha_beta)
  alpha-beta to ABC/1(Va) -> Scope1/1, Subsystem/1(Va)
  alpha-beta to ABC/2(Vb) -> Scope1/2, Subsystem/2(Vb)
  alpha-beta to ABC/3(Vc) -> Scope1/3, Subsystem/3(Vc)
  Demux1/5 -> g5/1
  Demux1/4 -> g6/1
  Demux1/2 -> g4/1
  Demux1/3 -> g3/1
  Subsystem/4(g6) -> Mux1/4  "g6"
  Subsystem/2(g4) -> Mux1/2  "g4"
  Subsystem/5(g5) -> Mux1/5  "g5"
  Demux1/1 -> g1/1
  Subsystem/6(g2) -> Mux1/6  "g2"
  Mux1/1 -> Demux1/1, Gate1/1
  Subsystem/3(g3) -> Mux1/3  "g3"
  Demux1/6 -> g2/1
  Subsystem/1(g1) -> Mux1/1  "g1"

== system NandiniG_23EEM1S02_bldc_foc/PWM generator/PWM/Gate Pulse ==
  gates : Inport
  Compare To Zero : simulink/Logic and Bit Operations/Compare To Zero  relop=>=  OutDataTypeStr=boolean
  Compare To Zero1 : simulink/Logic and Bit Operations/Compare To Zero  relop=>=  OutDataTypeStr=boolean
  Compare To Zero2 : simulink/Logic and Bit Operations/Compare To Zero  relop=>=  OutDataTypeStr=boolean
  Compare To Zero3 : simulink/Logic and Bit Operations/Compare To Zero  relop=<=  OutDataTypeStr=boolean
  Compare To Zero4 : simulink/Logic and Bit Operations/Compare To Zero  relop=<=  OutDataTypeStr=boolean
  Compare To Zero5 : simulink/Logic and Bit Operations/Compare To Zero  relop=<=  OutDataTypeStr=boolean
  Demux : Demux  Outputs=3
  Mux : Mux  Inputs=6
  Out1 : Outport
  wires:
  Compare To Zero1/1 -> Mux/3
  Demux/2 -> Compare To Zero4/1, Compare To Zero1/1
  Compare To Zero3/1 -> Mux/2
  Demux/3 -> Compare To Zero5/1, Compare To Zero2/1
  Compare To Zero2/1 -> Mux/5
  Demux/1 -> Compare To Zero3/1, Compare To Zero/1
  Compare To Zero4/1 -> Mux/4
  Compare To Zero5/1 -> Mux/6
  Compare To Zero/1 -> Mux/1
  gates/1 -> Demux/1
  Mux/1 -> Out1/1

== system NandiniG_23EEM1S02_bldc_foc/PWM generator/PWM/alpha-beta to ABC ==
  alpha_beta : Inport
  Demux : Demux  Outputs=2
  Gain5 : Gain  Gain=2/3
  Gain6 : Gain  Gain=1/sqrt(3)
  Gain7 : Gain  Gain=-1/3
  Gain8 : Gain  Gain=-1/3
  Gain9 : Gain  Gain=-1/sqrt(3)
  Sum1 : Sum  Inputs=|++
  Sum2 : Sum  Inputs=|++
  Va : Outport
  Vb : Outport  Port=2
  Vc : Outport  Port=3
  wires:
  Demux/1 -> Gain5/1, Gain8/1, Gain7/1
  Gain5/1 -> Va/1
  Demux/2 -> Gain9/1, Gain6/1
  Gain6/1 -> Sum1/1
  Gain7/1 -> Sum1/2
  Sum1/1 -> Vb/1
  Gain8/1 -> Sum2/1
  Gain9/1 -> Sum2/2
  Sum2/1 -> Vc/1
  alpha_beta/1 -> Demux/1

== system NandiniG_23EEM1S02_bldc_foc/PWM generator/SPWM/alpha-beta to ABC ==
  alpha_beta : Inport
  Demux : Demux  Outputs=2
  Gain5 : Gain  Gain=2/3
  Gain6 : Gain  Gain=1/sqrt(3)
  Gain7 : Gain  Gain=-1/3
  Gain8 : Gain  Gain=-1/3
  Gain9 : Gain  Gain=-1/sqrt(3)
  Sum1 : Sum  Inputs=|++
  Sum2 : Sum  Inputs=|++
  Va : Outport
  Vb : Outport  Port=2
  Vc : Outport  Port=3
  wires:
  Demux/1 -> Gain5/1, Gain8/1, Gain7/1
  Gain5/1 -> Va/1
  Demux/2 -> Gain9/1, Gain6/1
  Gain6/1 -> Sum1/1
  Gain7/1 -> Sum1/2
  Sum1/1 -> Vb/1
  Gain8/1 -> Sum2/1
  Gain9/1 -> Sum2/2
  Sum2/1 -> Vc/1
  alpha_beta/1 -> Demux/1

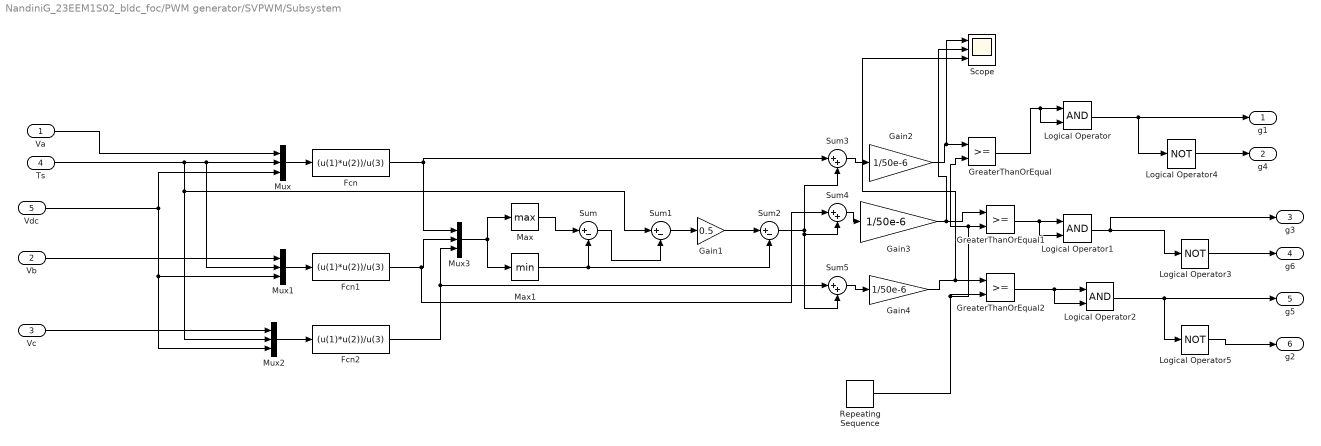
== system NandiniG_23EEM1S02_bldc_foc/PWM generator/SVPWM/Subsystem ==
  Va : Inport
  Vb : Inport  Port=2
  Vc : Inport  Port=3
  Ts : Inport  Port=4
  Vdc : Inport  Port=5
  Fcn : Fcn  Expr=(u(1)*u(2))/u(3)
  Fcn1 : Fcn  Expr=(u(1)*u(2))/u(3)
  Fcn2 : Fcn  Expr=(u(1)*u(2))/u(3)
  Gain1 : Gain  Gain=0.5
  Gain2 : Gain  Gain=1/50e-6
  Gain3 : Gain  Gain=1/50e-6
  Gain4 : Gain  Gain=1/50e-6
  GreaterThanOrEqual : RelationalOperator  OutDataTypeStr=boolean  RndMeth=Simplest  InputSameDT=off
  GreaterThanOrEqual1 : RelationalOperator  OutDataTypeStr=boolean  RndMeth=Simplest  InputSameDT=off
  GreaterThanOrEqual2 : RelationalOperator  OutDataTypeStr=boolean  RndMeth=Simplest  InputSameDT=off
  Logical Operator : Logic  AllPortsSameDT=off  OutDataTypeStr=boolean
  Logical Operator1 : Logic  AllPortsSameDT=off  OutDataTypeStr=boolean
  Logical Operator2 : Logic  AllPortsSameDT=off  OutDataTypeStr=boolean
  Logical Operator3 : Logic  Operator=NOT  AllPortsSameDT=off  OutDataTypeStr=boolean
  Logical Operator4 : Logic  Operator=NOT  AllPortsSameDT=off  OutDataTypeStr=boolean
  Logical Operator5 : Logic  Operator=NOT  AllPortsSameDT=off  OutDataTypeStr=boolean
  Max : MinMax  Function=max
  Max1 : MinMax
  Mux{,1..3} (4 alike) : Mux  Inputs=3
  Repeating Sequence : simulink/Sources/Repeating Sequence  rep_seq_t=[0 0.25 0.5 0.75 1]/1250  rep_seq_y=[1 0 -1 0 1]
  Scope : Scope  NumInputPorts=3
  Sum : Sum  Inputs=|+-
  Sum1 : Sum  Inputs=|+-
  Sum2 : Sum  Inputs=|+-
  Sum3 : Sum  Inputs=|++
  Sum4 : Sum  Inputs=|++
  Sum5 : Sum  Inputs=|++
  g1 : Outport
  g4 : Outport  Port=2
  g3 : Outport  Port=3
  g6 : Outport  Port=4
  g5 : Outport  Port=5
  g2 : Outport  Port=6
  wires:
  Ts/1 -> Sum1/1, Mux2/2, Mux1/2, Mux/2
  GreaterThanOrEqual1/1 -> Logical Operator1/2, Logical Operator1/1
  Sum2/1 -> Sum5/2, Sum4/2, Sum3/2
  Logical Operator1/1 -> Logical Operator3/1, g3/1
  Vdc/1 -> Mux/3, Mux1/3, Mux2/3
  Logical Operator4/1 -> g4/1
  Logical Operator2/1 -> g5/1, Logical Operator5/1
  Sum5/1 -> Gain4/1
  Repeating Sequence/1 -> GreaterThanOrEqual/2, GreaterThanOrEqual1/2, GreaterThanOrEqual2/2
  Logical Operator/1 -> g1/1, Logical Operator4/1
  Fcn/1 -> Sum3/1, Mux3/1
  Sum3/1 -> Gain2/1
  Gain4/1 -> Scope/3, GreaterThanOrEqual2/1
  Gain2/1 -> Scope/1, GreaterThanOrEqual/1
  Gain1/1 -> Sum2/1
  Mux3/1 -> Max/1, Max1/1
  Sum4/1 -> Gain3/1
  GreaterThanOrEqual/1 -> Logical Operator/2, Logical Operator/1
  Vb/1 -> Mux1/1
  Fcn2/1 -> Sum5/1, Mux3/3
  Fcn1/1 -> Sum4/1, Mux3/2
  Vc/1 -> Mux2/1
  GreaterThanOrEqual2/1 -> Logical Operator2/2, Logical Operator2/1
  Max/1 -> Sum/1
  Mux2/1 -> Fcn2/1
  Mux1/1 -> Fcn1/1
  Sum1/1 -> Gain1/1
  Mux/1 -> Fcn/1
  Va/1 -> Mux/1
  Max1/1 -> Sum2/2, Sum/2
  Sum/1 -> Sum1/2
  Gain3/1 -> Scope/2, GreaterThanOrEqual1/1
  Logical Operator3/1 -> g6/1
  Logical Operator5/1 -> g2/1

== system NandiniG_23EEM1S02_bldc_foc/PWM generator/SVPWM/Subsystem1 ==
  alpha beta : Inport
  Demux : Demux  Commented=on  Outputs=6
  Mux4 : Mux  Commented=on  Inputs=6
  Space Vector PWM : Subsystem  Commented=on
  Out1 : Outport
  Out2 : Outport  Port=2
  Out3 : Outport  Port=3
  Out4 : Outport  Port=4
  Out5 : Outport  Port=5
  Out6 : Outport  Port=6
  wires:
  Space Vector PWM/6(Vg2) -> Mux4/6  "g2"
  Mux4/1 -> Demux/1
  Demux/1 -> Out1/1
  Space Vector PWM/1(Vg1) -> Mux4/1  "g1"
  Space Vector PWM/3(Vg3) -> Mux4/3  "g3"
  Space Vector PWM/4(Vg6) -> Mux4/4  "g6"
  Space Vector PWM/2(Vg4) -> Mux4/2  "g4"
  alpha beta/1 -> Space Vector PWM/1(alpha beta)
  Demux/3 -> Out3/1
  Space Vector PWM/5(Vg5) -> Mux4/5  "g5"
  Demux/2 -> Out2/1
  Demux/5 -> Out5/1
  Demux/4 -> Out4/1
  Demux/6 -> Out6/1

== system NandiniG_23EEM1S02_bldc_foc/PWM generator/SVPWM/alpha-beta to ABC ==
  alpha_beta : Inport
  Demux : Demux  Outputs=2
  Gain5 : Gain  Gain=2/3
  Gain6 : Gain  Gain=1/sqrt(3)
  Gain7 : Gain  Gain=-1/3
  Gain8 : Gain  Gain=-1/3
  Gain9 : Gain  Gain=-1/sqrt(3)
  Scope : Scope  NumInputPorts=3
  Sum1 : Sum  Inputs=|++
  Sum2 : Sum  Inputs=|++
  Va : Outport
  Vb : Outport  Port=2
  Vc : Outport  Port=3
  wires:
  Demux/1 -> Gain5/1, Gain8/1, Gain7/1
  Gain5/1 -> Scope/1, Va/1
  Demux/2 -> Gain9/1, Gain6/1
  Gain6/1 -> Sum1/1
  Gain7/1 -> Sum1/2
  Sum1/1 -> Scope/2, Vb/1
  Gain8/1 -> Sum2/1
  Gain9/1 -> Sum2/2
  Sum2/1 -> Scope/3, Vc/1
  alpha_beta/1 -> Demux/1

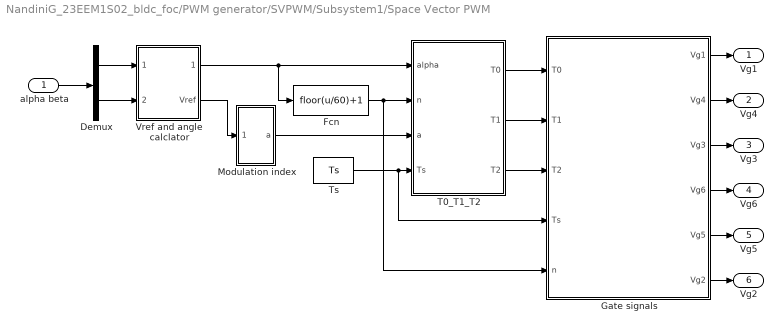
== system NandiniG_23EEM1S02_bldc_foc/PWM generator/SVPWM/Subsystem1/Space Vector PWM ==
  alpha beta : Inport
  Demux : Demux  Outputs=2
  Fcn : Fcn  Expr=floor(u/60)+1
  Gate signals : Subsystem
  Modulation index : Subsystem
  T0_T1_T2 : Subsystem
  Ts : Constant  Value=Ts
  Vref and angle calclator : Subsystem
  Vg1 : Outport  VectorParamsAs1DForOutWhenUnconnected=off
  Vg4 : Outport  Port=2  VectorParamsAs1DForOutWhenUnconnected=off
  Vg3 : Outport  Port=3  VectorParamsAs1DForOutWhenUnconnected=off
  Vg6 : Outport  Port=4  VectorParamsAs1DForOutWhenUnconnected=off
  Vg5 : Outport  Port=5  VectorParamsAs1DForOutWhenUnconnected=off
  Vg2 : Outport  Port=6  VectorParamsAs1DForOutWhenUnconnected=off
  wires:
  Fcn/1 -> T0_T1_T2/2(n), Gate signals/5(n)
  T0_T1_T2/3(T2) -> Gate signals/3(T2)
  Demux/2 -> Vref and angle calclator/2(Vbeta)
  Gate signals/5(Vg5) -> Vg5/1
  Gate signals/4(Vg6) -> Vg6/1
  Gate signals/2(Vg4) -> Vg4/1
  Gate signals/3(Vg3) -> Vg3/1
  Gate signals/1(Vg1) -> Vg1/1
  Ts/1 -> Gate signals/4(Ts), T0_T1_T2/4(Ts)
  Gate signals/6(Vg2) -> Vg2/1
  T0_T1_T2/1(T0) -> Gate signals/1(T0)
  T0_T1_T2/2(T1) -> Gate signals/2(T1)
  Vref and angle calclator/2(Vref) -> Modulation index/1(Vref)
  Modulation index/1(a) -> T0_T1_T2/3(a)
  Vref and angle calclator/1(alpha) -> Fcn/1, T0_T1_T2/1(alpha)
  alpha beta/1 -> Demux/1
  Demux/1 -> Vref and angle calclator/1(Valpha)

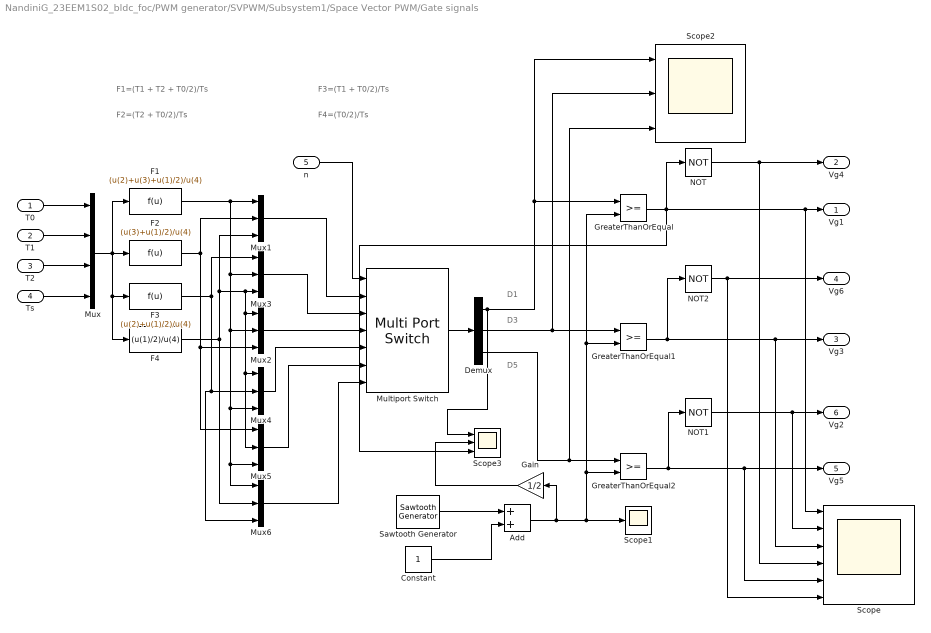
== system NandiniG_23EEM1S02_bldc_foc/PWM generator/SVPWM/Subsystem1/Space Vector PWM/Gate signals ==
  note: D1
  note: F1=(T1 + T2 + T0/2)/Ts
  note: F2=(T2 + T0/2)/Ts
  note: F3=(T1 + T0/2)/Ts
  note: F4=(T0/2)/Ts
  note: D3
  note: D5
  T0 : Inport
  T1 : Inport  Port=2
  T2 : Inport  Port=3
  Ts : Inport  Port=4
  n : Inport  Port=5
  Add : Sum
  Constant : Constant
  Demux : Demux  Outputs=3
  F1 : Fcn  Expr=(u(2)+u(3)+u(1)/2)/u(4)
  F2 : Fcn  Expr=(u(3)+u(1)/2)/u(4)
  F3 : Fcn  Expr=(u(2)+u(1)/2)/u(4)
  F4 : Fcn  Expr=(u(1)/2)/u(4)
  Gain : Gain  Gain=1/2
  GreaterThanOrEqual : RelationalOperator  OutDataTypeStr=boolean  RndMeth=Simplest  InputSameDT=off
  GreaterThanOrEqual1 : RelationalOperator  OutDataTypeStr=boolean  RndMeth=Simplest  InputSameDT=off
  GreaterThanOrEqual2 : RelationalOperator  OutDataTypeStr=boolean  RndMeth=Simplest  InputSameDT=off
  Multiport Switch : MultiPortSwitch  Inputs=6  DiagnosticForDefault=None  SaturateOnIntegerOverflow=off  InputSameDT=off
  Mux : Mux
  Mux{1..6} (6 alike) : Mux  Inputs=3
  NOT : Logic  Operator=NOT  IconShape=distinctive  AllPortsSameDT=off  OutDataTypeStr=boolean
  NOT1 : Logic  Operator=NOT  IconShape=distinctive  AllPortsSameDT=off  OutDataTypeStr=boolean
  NOT2 : Logic  Operator=NOT  IconShape=distinctive  AllPortsSameDT=off  OutDataTypeStr=boolean
  Sawtooth Generator : spsSawtoothGeneratorLib/Sawtooth Generator  Freq=5e3  Phase=0  Ts=0
  Scope : Scope  NumInputPorts=6
  Scope1 : Scope
  Scope2 : Scope  NumInputPorts=3
  Scope3 : Scope  NumInputPorts=3
  Vg1 : Outport  VectorParamsAs1DForOutWhenUnconnected=off
  Vg4 : Outport  Port=2  VectorParamsAs1DForOutWhenUnconnected=off
  Vg3 : Outport  Port=3  VectorParamsAs1DForOutWhenUnconnected=off
  Vg6 : Outport  Port=4  VectorParamsAs1DForOutWhenUnconnected=off
  Vg5 : Outport  Port=5  VectorParamsAs1DForOutWhenUnconnected=off
  Vg2 : Outport  Port=6  VectorParamsAs1DForOutWhenUnconnected=off
  wires:
  Demux/2 -> GreaterThanOrEqual1/1, Scope2/2
  Sawtooth Generator/1 -> Add/1
  GreaterThanOrEqual/1 -> Scope3/3, Scope/1, Vg1/1, NOT/1
  GreaterThanOrEqual1/1 -> NOT2/1, Scope/3, Vg3/1
  GreaterThanOrEqual2/1 -> NOT1/1, Scope/5, Vg5/1
  NOT/1 -> Scope/4, Vg4/1
  NOT1/1 -> Scope/2, Vg2/1
  NOT2/1 -> Scope/6, Vg6/1
  n/1 -> Multiport Switch/1
  T0/1 -> Mux/1
  T1/1 -> Mux/2
  T2/1 -> Mux/3
  Ts/1 -> Mux/4
  Mux/1 -> F1/1, F2/1, F4/1, F3/1
  Demux/3 -> GreaterThanOrEqual2/1, Scope2/3
  Add/1 -> Gain/1, Scope1/1, GreaterThanOrEqual2/2, GreaterThanOrEqual1/2, GreaterThanOrEqual/2
  Constant/1 -> Add/2
  Multiport Switch/1 -> Demux/1
  Demux/1 -> Scope3/1, GreaterThanOrEqual/1, Scope2/1
  Mux6/1 -> Multiport Switch/7
  Mux5/1 -> Multiport Switch/6
  Mux4/1 -> Multiport Switch/5
  Mux2/1 -> Multiport Switch/4
  Mux3/1 -> Multiport Switch/3
  Mux1/1 -> Multiport Switch/2
  F1/1 -> Mux6/1, Mux5/3, Mux4/3, Mux2/2, Mux3/2, Mux1/1
  F2/1 -> Mux1/2, Mux5/1, Mux2/3
  F4/1 -> Mux6/2, Mux5/2, Mux4/1, Mux2/1, Mux3/3, Mux1/3
  F3/1 -> Mux6/3, Mux4/2, Mux3/1
  Gain/1 -> Scope3/2

== system NandiniG_23EEM1S02_bldc_foc/PWM generator/SVPWM/Subsystem1/Space Vector PWM/Modulation index ==
  Vref : Inport
  Abs : Abs  SaturateOnIntegerOverflow=off
  Fcn1 : Fcn  Expr=u(1)/((2/3)*u(2))
  M1 : Constant  Value=0.86
  Mux : Mux  Inputs=2
  Scope : Scope
  Switch : Switch  Threshold=0.866  SaturateOnIntegerOverflow=off  InputSameDT=off
  Vs : Constant  Value=106.67
  a : Outport  VectorParamsAs1DForOutWhenUnconnected=off
  wires:
  Fcn1/1 -> Switch/3, Switch/2
  Vs/1 -> Mux/2
  M1/1 -> Switch/1
  Vref/1 -> Abs/1
  Mux/1 -> Fcn1/1
  Switch/1 -> Scope/1, a/1
  Abs/1 -> Mux/1

== system NandiniG_23EEM1S02_bldc_foc/PWM generator/SVPWM/Subsystem1/Space Vector PWM/T0_T1_T2 ==
  alpha : Inport
  n : Inport  Port=2
  a : Inport  Port=3
  Ts : Inport  Port=4
  Mux : Mux
  Scope1 : Scope  NumInputPorts=3
  Sum : Sum  Inputs=|--+
  T_1 : Fcn  Expr=(u(3)*u(4)*(sin((u(2)*pi/3)-u(1)*pi/180)))/(sin(pi/3))
  T_2 : Fcn  Expr=(u(3)*u(4)*(sin(u(1)*pi/180-((u(2)-1)*pi/3))))/(sin(pi/3))
  T0 : Outport  VectorParamsAs1DForOutWhenUnconnected=off
  T1 : Outport  Port=2  VectorParamsAs1DForOutWhenUnconnected=off
  T2 : Outport  Port=3  VectorParamsAs1DForOutWhenUnconnected=off
  wires:
  Mux/1 -> T_2/1, T_1/1
  n/1 -> Mux/2
  a/1 -> Mux/3
  Ts/1 -> Sum/3, Mux/4
  T_2/1 -> Sum/2, Scope1/3, T2/1
  T_1/1 -> Scope1/1, T1/1, Sum/1
  Sum/1 -> Scope1/2, T0/1
  alpha/1 -> Mux/1

== system NandiniG_23EEM1S02_bldc_foc/PWM generator/SVPWM/Subsystem1/Space Vector PWM/Vref and angle calclator ==
  Valpha : Inport
  Vbeta : Inport  Port=2
  Complex to Magnitude-Angle : ComplexToMagnitudeAngle
  Real-Imag to Complex : RealImagToComplex
  rad to deg : Subsystem
  alpha : Outport  VectorParamsAs1DForOutWhenUnconnected=off
  Vref : Outport  Port=2  VectorParamsAs1DForOutWhenUnconnected=off
  wires:
  Valpha/1 -> Real-Imag to Complex/1
  Real-Imag to Complex/1 -> Complex to Magnitude-Angle/1
  Vbeta/1 -> Real-Imag to Complex/2
  rad to deg/1(2D) -> alpha/1
  Complex to Magnitude-Angle/2 -> rad to deg/1(R)
  Complex to Magnitude-Angle/1 -> Vref/1

== system NandiniG_23EEM1S02_bldc_foc/PWM generator/SVPWM/Subsystem1/Space Vector PWM/Vref and angle calclator/rad to deg ==
  R : Inport
  Constant1 : Constant  Value=2*pi
  Radians to Degrees1 : simulink_extras/Transformations/Radians to Degrees
  Sum : Sum  Inputs=|++
  Switch : Switch  SaturateOnIntegerOverflow=off  InputSameDT=off
  2D : Outport  VectorParamsAs1DForOutWhenUnconnected=off
  wires:
  R/1 -> Switch/2, Switch/1, Sum/1
  Radians to Degrees1/1 -> 2D/1
  Switch/1 -> Radians to Degrees1/1
  Sum/1 -> Switch/3
  Constant1/1 -> Sum/2
